simulink model "simli_wdc_wWT"  (R2023b)
settings: Solver=VariableStepAuto  StartTime=0.0  StopTime=10  RelTol=1e-3
undefined symbols (not defined in the file or in its folder): A_s_denom, A_s_num, c_f, C_hv_km, Cagg, Cbase1v, Cbase_hv, Cbase_mv, delta_vsc_0, G_dc_denom, G_dc_num, H_gen, H_vsm, i_d_vsc, i_q_vsc, Ibase_hv, Ibase_mv, k_d_vsm, k_p_p_vsm, k_p_q_vsm, k_vc, ki, ki_q, kp, L_comp, l_f, l_grid, L_hv_km, l_t_ehvhv, l_t_hvmv, l_t_mvlv, Lagg, Lbase_hv, Lbase_mv, length_export, M_gr_denom, M_gr_num, mppt_gain, omega_nom, omega_WTR_0, omega_WTR_n, P_meas, P_t, phase_shift_test_state, phase_shifts, pie_export, Q_meas, r_f, r_grid, R_hv_km, r_sys, r_t_ehvhv, r_t_hvmv, r_t_mvlv, Ragg, Rd, rocof_slope, Rocof_test_state, T_dc_denom, T_dc_num ... (+21)
libraries: slpidlib x9, spsFirstOrderFilterLib x1, simulink x1, spsSampleandHoldLib x1, spspowerguiLib x1
(part 1 of 3)
settings Model: Creator=Martin Pedersen  LastModifiedBy=Martin Pedersen

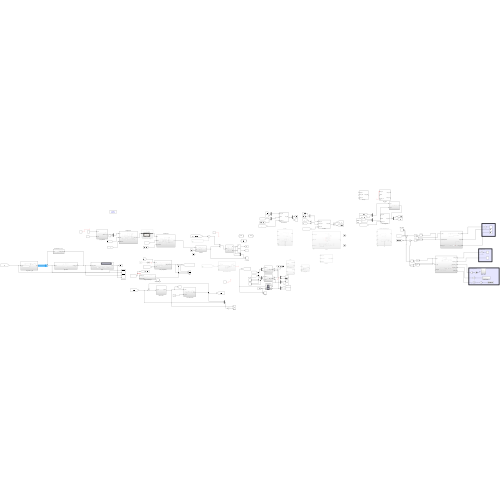
[thumbnail: Simulink's stored preview of the top-level diagram]
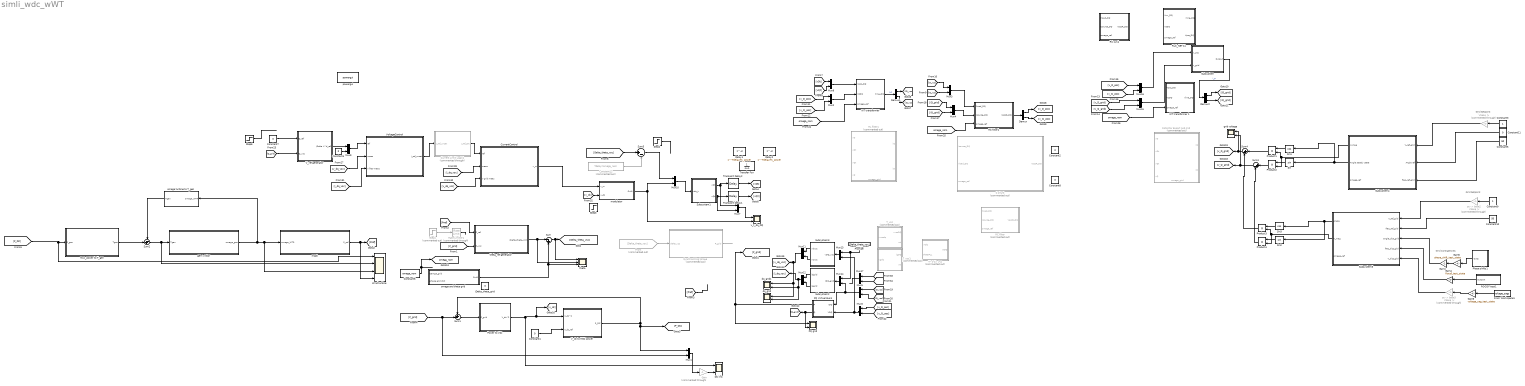
== system simli_wdc_wWT ==
  note: Grid Setpoint
  note: Grid Setpoint
  note: Grid Contigencies
  C shunt : Subsystem  Commented=on
  Collector Export and grid : Subsystem  Commented=on
      settings: PortSchema="{\"entries\":[{\"content\":{\"sides\":[{\"content\":{\"connectorIds\":[\"In1\",\"In2\",\"In3\",\"In4\"]},\"type\":\"ConnectorPlacement.EquallySpacedRectSide\",\"uuid\":\"57ad71d1-5664-4b35-a20c-d71f7e1cdc47\"},{\"content\":{\"connectorIds\":[\"Out1\",\"Out2\"],\"side\":\"RIGHT\"},\"type\":\"ConnectorPlacement.EquallySpacedRectSide\",\"uuid\":\"8101605d-eedb-4c26-847d-0cc0ce629d60\"},{\"content\":{\"side\":\"TOP\"},\"type\":\"ConnectorPlacement.EquallySpacedRectSide\",\"uuid\":\"2627b00b-24a5-469a-be2d-9c3c8a1d2080\"},{\"content\":{\"connectorIds\":[\"In5\"],\"side\":\"BOTTOM\"},\"type\":\"ConnectorPlacement.EquallySpacedRectSide\",\"uuid\":\"fe553db7-7727-4a02-b1e7-5aedfb7840ee\"}]},\"type\":\"ConnectorPlacement.EquallySpacedConnector\",\"uuid\":\"f40200c8-ad5b-428c-8a4e-7641595b86c4\"}],\"packageUris\":[\"http://schema.mathworks.com/mf0/Connector/R2020b\"],\"version\":\"1.0\"}"
  Constant{1..2,7..8,11} (5 alike) : Constant  Value=0
  Constant10 : Constant  Value=50
  Constant12 : Constant  Commented=on  Value=Tdelay*omega_nom
  Constant3 : Constant
  Constant4 : Constant  Value=0  SampleTime=Ts_power
  Constant5 : Constant  Value=50
  Constant6 : Constant  Value=omega_nom
  Constant9 : Constant
  Current Limit Logic1 : Subsystem  Commented=through
  CurrentControl : Subsystem
  DC link : Scope  NumInputPorts=2
  Delay1 : Delay  DelayLength=Tdelay/Ts_power
  Delay2 : Delay  DelayLength=Tdelay/Ts_power
  Demux : Demux  Outputs=2
  Demux1 : Demux  Outputs=2
  Demux2 : Demux  Outputs=2
  From : From  Commented=on  GotoTag=Delta_theta_vsc
  From Workspace1 : FromWorkspace  VariableName=voltage_sags
  Gain : Gain  Commented=through  Gain=-1
  Gain1 : Gain  Gain=-1
  Gain4 : Gain  Gain=Rocof_test_state
  Gain5 : Gain  Gain=phase_shift_test_state
  Gain6 : Gain  Gain=voltage_sag_test_state
  Mux{1..17} (17 alike) : Mux  Inputs=2
  PQ Virtual Bus1 : Subsystem
  PQ grid : Scope  NumInputPorts=2
  Phase shifts1 : Subsystem
  Power to Vdc : Subsystem
  Product{1..4} (4 alike) : Product
  RC filter : Subsystem  Commented=on  mask{Csource=c_f/omega_nom, Rd=0, VD0=1, VQ0=0}
      mask prompts: Csource "Net Capacitance"; Rd "Rdamp"
      mask help:
      | PI network, capacitance to enter is total.
      | Left and right current as input. Left and right voltage as output
      mask init:
      | inv_Csource=1/Csource;
      mask TypeOptions Csource: 8/Gain
      mask TypeOptions Rd: 1/Gain | 2/Gain
      mask TypeOptions VD0: VcpdR_int/InitialCondition
      mask TypeOptions VQ0: VcpqR_int/InitialCondition
  RC filter1 : Subsystem  mask{Csource=(c_f)/omega_nom, Rd=0, VD0=0, VQ0=0}
      mask prompts: Csource "Net Capacitance"; Rd "Rdamp"
      mask help:
      | PI network, capacitance to enter is total.
      | Left and right current as input. Left and right voltage as output
      mask init:
      | inv_Csource=1/Csource;
      mask TypeOptions Csource: 8/Gain
      mask TypeOptions Rd: 1/Gain | 2/Gain
      mask TypeOptions VD0: VcpdR_int/InitialCondition
      mask TypeOptions VQ0: VcpqR_int/InitialCondition
  RC sys1 : Subsystem  mask{Csource=(C_hv_km*length_export/Cbase_hv)/omega_nom, Rd=0.0001, VD0=0, VQ0=0}
      mask prompts: Csource "Net Capacitance"; Rd "Rdamp"
      mask help:
      | PI network, capacitance to enter is total.
      | Left and right current as input. Left and right voltage as output
      mask init:
      | inv_Csource=1/Csource;
      mask TypeOptions Csource: 8/Gain
      mask TypeOptions Rd: 1/Gain | 2/Gain
      mask TypeOptions VD0: VcpdR_int/InitialCondition
      mask TypeOptions VQ0: VcpqR_int/InitialCondition
  RL filter1 : Subsystem  Commented=on
      settings: PortSchema="{\"entries\":[{\"content\":{\"sides\":[{\"content\":{\"connectorIds\":[\"In1\",\"In2\",\"In3\",\"In4\"]},\"type\":\"ConnectorPlacement.EquallySpacedRectSide\",\"uuid\":\"57ad71d1-5664-4b35-a20c-d71f7e1cdc47\"},{\"content\":{\"connectorIds\":[\"Out1\",\"Out2\"],\"side\":\"RIGHT\"},\"type\":\"ConnectorPlacement.EquallySpacedRectSide\",\"uuid\":\"8101605d-eedb-4c26-847d-0cc0ce629d60\"},{\"content\":{\"side\":\"TOP\"},\"type\":\"ConnectorPlacement.EquallySpacedRectSide\",\"uuid\":\"2627b00b-24a5-469a-be2d-9c3c8a1d2080\"},{\"content\":{\"connectorIds\":[\"In5\"],\"side\":\"BOTTOM\"},\"type\":\"ConnectorPlacement.EquallySpacedRectSide\",\"uuid\":\"fe553db7-7727-4a02-b1e7-5aedfb7840ee\"}]},\"type\":\"ConnectorPlacement.EquallySpacedConnector\",\"uuid\":\"f40200c8-ad5b-428c-8a4e-7641595b86c4\"}],\"packageUris\":[\"http://schema.mathworks.com/mf0/Connector/R2020b\"],\"version\":\"1.0\"}"
  RLC_NET 11 : Subsystem  mask{Csource=(C_hv_km*length_export/pie_export/Cbase_hv)/omega_nom, Rsource=(R_hv_km*length_export/pie_export)/Zbase_hv, Lsource=(L_hv_km*length_export/pie_export/Lbase_hv)/omega_nom}
      mask prompts: Csource "line capacitance 1 side"; Rsource "Line resistance"; Lsource "line inductance"
      mask help:
      | RL with C terminations on right,
      | Left Voltage  and Right current input, Right voltage and left current output
      mask init:
      | inv_Csource=1/Csource;
      | inv_Lsource=1/Lsource;
      mask TypeOptions Csource: 8/Gain
      mask TypeOptions Rsource: 2/Gain | 3/Gain
      mask TypeOptions Lsource: 7/Gain
  ROCOF test1 : Subsystem
  Rate Limiter1 : RateLimiter  Commented=through  SampleTimeMode=inherited
  Sin : Trigonometry
  Sin1 : Trigonometry  Operator=cos
  Sin2 : Trigonometry
  Sin3 : Trigonometry  Operator=cos
  Step1 : Step  Commented=on  After=0.1  SampleTime=Ts_power
  Step2 : Step  Time=5  After=0  SampleTime=Ts_power
  Step3 : Step  Time=5  After=0  SampleTime=Ts_power
  Step6 : Step  After=0.1  SampleTime=Ts_power
  Subsystem : Subsystem
  Subsystem1 : Subsystem
  Subsystem2 : Subsystem
  Subsystem3 : Subsystem
  Subsystem4 : Subsystem
  Subsystem5 : Subsystem
  Sum : Sum  Inputs=|-+
  Sum1 : Sum  Inputs=+-|
  Sum2 : Sum  Inputs=-+|
  Sum3 : Sum  Inputs=|+-
  Sum4 : Sum  Inputs=|+-
  Sum5 : Sum  Inputs=|+-
  Synchronizing torque : Subsystem  Commented=on
  "T^{-1}_vsc" : Subsystem  Commented=on
  T_vsc : Subsystem  Commented=on  AncestorBlock=powerlib_meascontrol/Transformations/dq0 to Alpha-Beta-Zero/Subsystem1
  T_vsc1 : Subsystem  Commented=on  AncestorBlock=powerlib_meascontrol/Transformations/dq0 to Alpha-Beta-Zero/Subsystem1
  Transfer Fcn : TransferFcn  Denominator=[1 1]
  Transport Delay1 : TransportDelay  DelayTime=Tdelay/4  BufferSize=3560000  TransDelayFeedthrough=on
  Transport Delay2 : TransportDelay  DelayTime=Tdelay/4  BufferSize=3560000  TransDelayFeedthrough=on
  V_dc to MSC power : Subsystem
  V_ref generator : Subsystem
  VoltageControl : Subsystem
  "WT transformer " : Subsystem  mask{Rsource=r_f, Lsource=l_f/omega_nom}
      mask prompts: Rsource "Line resistance"; Lsource "line inductance"
      mask help:
      | RLV_NET is an 3 phase series RL with no virtual resistance termination,
      | 2 voltages as inputs and 1 current output
      mask init:
      | inv_Lsource=1/Lsource;
      mask TypeOptions Rsource: 2/Gain | 3/Gain
      mask TypeOptions Lsource: 7/Gain
  WT transformer 1 : Subsystem  mask{Rsource=r_sys, Lsource=x_sys/omega_nom}
      mask prompts: Rsource "Line resistance"; Lsource "line inductance"
      mask help:
      | RLV_NET is an 3 phase series RL with no virtual resistance termination,
      | 2 voltages as inputs and 1 current output
      mask init:
      | inv_Lsource=1/Lsource;
      mask TypeOptions Rsource: 2/Gain | 3/Gain
      mask TypeOptions Lsource: 7/Gain
  Wind turbine : Scope  NumInputPorts=4
  \Delta_theta_grid : Constant  Value=0
  dq_grid : Scope  NumInputPorts=2
  dq_grid1 : Scope  NumInputPorts=2
  gen->rotor : Subsystem
  grid voltage : Scope  NumInputPorts=2
  modulator : Subsystem
  mppt : Subsystem
  msc_power to T_gen : Subsystem
  omega and theta grid : Subsystem
  omega turbine to T_gen : Subsystem
  powergui : spspowerguiLib/powergui  Priority=1  SimulationMode=Discrete  SampleTime=Ts_power  frequency=60  Iterations=50  frequencyindice=60  Pbase=100e6  ErrMax=1e-4  UnitsV=kV  UnitsW=MW  buscounter=0  FunctionMessages=off  echomessages=off  EnableUseOfTLC=off  CurrentSourceSwitches=off  DisableSnubberDevices=off  DisableRonSwitches=off  DisableVfSwitches=off  DisplayEquations=off  AutomaticDiscreteSolvers=off  SolverType=Tustin/Backward Euler (TBE)  Interpol=off  ExternalGateDelay=off  methode=off  Ts=100  x0status=blocks  SPID=on  SwTol=0  HookPort=off  NonlinearTolerance=1e-4  nMaxIteration=100  ContinueOnMaxIteration=off  RestoreLinks=warning  ResistiveCurrentMeasurement=off  Frange=[0:2:500]  Ylog=off  Xlog=on  ShowGrid=off  save=off  variable=ZData  structure=0  ZoomFFT=off  StartTime=0.0  cycles=1  DisplayStyle=1  fundamental=60  FreqAxis=off  MaxFrequency=1000  frequencyindicesteady=1  RmsSteady=1  display=off
  "pu -> base" : Gain  Commented=through  Gain=Vbase_lv
  "pu -> base2" : Gain  Commented=through  Gain=Vbase_lv
  "pu -> base3" : Gain  Commented=through  Gain=Vbase_lv
  theta : Scope  NumInputPorts=3
  theta_ref generator : Subsystem
  v_t_dq_DQ : Scope  NumInputPorts=2
  tag scope: omega_nom=global
  wires:
  theta_ref generator/1(\Delta_theta_vsm) -> theta/2, Sum/1
  omega and theta grid/1(Out1) -> Sum/2, theta/3
  Sum/1 -> theta/1, [Delta_theta_vsc]
  V_ref generator/1(\Delta V^d_ref) -> Mux9/1
  From/1 -> Synchronizing torque/1(delta_vsc)
  [P_grid] -> theta_ref generator/2(P_vsc)
  [Pref] -> theta_ref generator/1(P_ref)
  [Pref] -> ?
  gen->rotor/1(omega_gen) -> omega turbine to T_gen/1(omega_WTR), Wind turbine/3, mppt/1(omega_WTR)
  Power to Vdc/1(V_dc^2) -> [v_dc], V_dc to MSC power/1(V_dc^2), DC link/1
  V_dc to MSC power/1(P_DC) -> Mux1/1, [P_DC], Sum1/1
  Sum1/1 -> Power to Vdc/1(P_grid)
  [P_grid] -> Mux1/2, Sum1/2
  Mux1/1 -> Gain/1
  Sum2/1 -> Wind turbine/2, gen->rotor/1(Tgen)
  msc_power to T_gen/1(Tgen) -> Sum2/2
  omega turbine to T_gen/1(Tgen) -> Sum2/1
  [P_DC] -> Wind turbine/1, msc_power to T_gen/1(P_gen)
  mppt/1(P_ref) -> Wind turbine/4, [Pref]
  Constant1/1 -> V_dc to MSC power/2(V_dc_ref)
  Step1/1 -> Rate Limiter1/1
  Gain/1 -> DC link/2
  Step2/1 -> ?
  Mux10/1 -> Subsystem1/1(vdq_t)
  [omega_nom] -> "WT transformer "/3(omega_ref)
  [vDt] -> Mux8/1
  [vQt] -> Mux8/2
  Demux1/1 -> [iD_vsc]
  Demux1/2 -> [iQ_vsc]
  [iQ_vsc] -> Mux3/2
  [iD_vsc] -> Mux3/1
  RC filter1/1(VpccR_DQ) -> Demux/1
  Demux/1 -> [v_D_poc]
  Demux/2 -> [v_Q_poc]
  [v_D_poc] -> Mux2/1
  [v_Q_poc] -> Mux2/2
  [v_Q_grid] -> Mux15/2
  [v_D_grid] -> Mux15/1
  Demux2/2 -> [iQ_grid]
  Demux2/1 -> [iD_grid]
  [v_Q_poc] -> Mux16/2
  [v_D_poc] -> Mux16/1
  [omega_nom] -> WT transformer 1/3(omega_ref)
  [iQ_grid] -> Mux4/2
  [iD_grid] -> Mux4/1
  [iQ_vsc] -> Mux5/2
  [iD_vsc] -> Mux5/1
  [v_Q_poc] -> Mux6/2
  [v_D_poc] -> Mux6/1
  PQ Virtual Bus1/2(Q) -> PQ grid/2, [Q_grid]
  [Q_grid] -> V_ref generator/2(Q_vsc)
  Step6/1 -> ?
  Mux7/1 -> v_t_dq_DQ/1
  [Delta_theta_vsc] -> Sum5/1
  Mux6/1 -> Mux13/2, PQ Virtual Bus1/2(VDQ)
  Mux4/1 -> RC filter1/2("Isource_DQ ")
  Mux3/1 -> RC filter1/1(Iload_DQ)
  [omega_nom] -> RC filter1/3(omega_ref)
  Constant6/1 -> [omega_nom]
  Synchronizing torque/1(P_grid) -> ?
  Rate Limiter1/1 -> ?
  VoltageControl/1(I_ref_unsat) -> Current Limit Logic1/1(I_ref_unsat)
  Current Limit Logic1/1(I_ref_sat) -> CurrentControl/1(ref)
  Constant4/1 -> Mux9/2
  Mux9/1 -> VoltageControl/1(ref)
  Mux5/1 -> Mux14/2, PQ Virtual Bus1/1(IDQ)
  Subsystem3/1(vdvsc) -> Mux11/1
  Subsystem3/2(vqvsc) -> Mux11/2
  Subsystem2/1(idgrid) -> Mux12/1
  Subsystem2/2(iqgrid) -> Mux12/2
  Mux12/1 -> dq_grid1/2, dq_grid/2, [i_dq_vsc]
  Mux11/1 -> dq_grid1/1, dq_grid/1, [v_dq_vsc]
  [v_dq_vsc] -> VoltageControl/2(meas)
  [i_dq_vsc] -> CurrentControl/2(meas)
  Mux14/1 -> Subsystem2/1(iDQ_grid)
  Mux13/1 -> Subsystem3/1(vDQ_vsc)
  [Delta_theta_vsc] -> Mux14/1, Mux13/1
  [v_dq_vsc] -> CurrentControl/3(V grid meas)
  [i_dq_vsc] -> VoltageControl/3(I filter meas)
  Constant7/1 -> V_ref generator/1(Q_ref)
  Mux2/1 -> "WT transformer "/2("VsDQ ")
  Mux8/1 -> "WT transformer "/1(Vpcc_DQ)
  "WT transformer "/1(Iline_DQ) -> Demux1/1  "i_o"
  Mux15/1 -> Subsystem/2(v_grid)
  Mux16/1 -> Subsystem/1(v_pcc)
  Subsystem/1(Output) -> Demux2/1  "i_o"
  [v_dc] -> modulator/2(v_dc)
  modulator/1(Out1) -> Mux10/2, v_t_dq_DQ/2
  Subsystem4/2(Angle steady state) -> Sin1/1, Sin/1
  "pu -> base"/1 -> Subsystem4/1(V_ref_grid)
  Sin1/1 -> Product1/1
  Sin2/1 -> Product4/1
  Subsystem4/1(V_mag) -> Product1/2, Product2/2
  Product3/1 -> Sum4/2
  From Workspace1/1 -> Gain6/1
  Gain4/1 -> Subsystem5/4(freq_dist_grid)
  Subsystem5/1(Angle) -> Sin2/1, Sin3/1
  Sum3/1 -> [v_Q_grid], grid voltage/2
  Gain1/1 -> Subsystem5/3(angle_dist_grid)
  Gain6/1 -> "pu -> base3"/1
  Constant9/1 -> "pu -> base2"/1
  "pu -> base2"/1 -> Subsystem5/1(V_ref_grid)
  ROCOF test1/1(Outport) -> Gain4/1
  Sin3/1 -> Product3/1
  Sin/1 -> Product2/1
  "pu -> base3"/1 -> Subsystem5/5(V_dist_grid)
  Subsystem5/2(V_mag) -> Product4/2, Product3/2
  Product2/1 -> Sum3/1
  Constant5/1 -> Subsystem4/3(freq_ref_grid)
  Constant10/1 -> Subsystem5/2(freq_ref_grid)
  Product1/1 -> Sum4/1
  Product4/1 -> Sum3/2
  Constant11/1 -> Subsystem4/2(Angle ref)
  Gain5/1 -> Gain1/1
  Phase shifts1/1(Out2) -> Gain5/1
  Sum4/1 -> grid voltage/1, [v_D_grid]
  Constant3/1 -> "pu -> base"/1
  Subsystem1/1(vDt) -> Transport Delay2/1, Mux7/1
  Subsystem1/2(vQt) -> Transport Delay1/1, Mux7/2
  Constant12/1 -> Sum5/2
  Sum5/1 -> Mux10/1
  CurrentControl/1(v_m) -> modulator/1(v_m)
  Transport Delay2/1 -> [vDt]
  Transport Delay1/1 -> [vQt]
  ? -> RLC_NET 11/1(Iinv_DQ)
  PQ Virtual Bus1/1(P) -> [P_grid], PQ grid/1
  Mux17/1 -> ?
  [iD_grid] -> Mux17/1
  [iQ_grid] -> Mux17/2

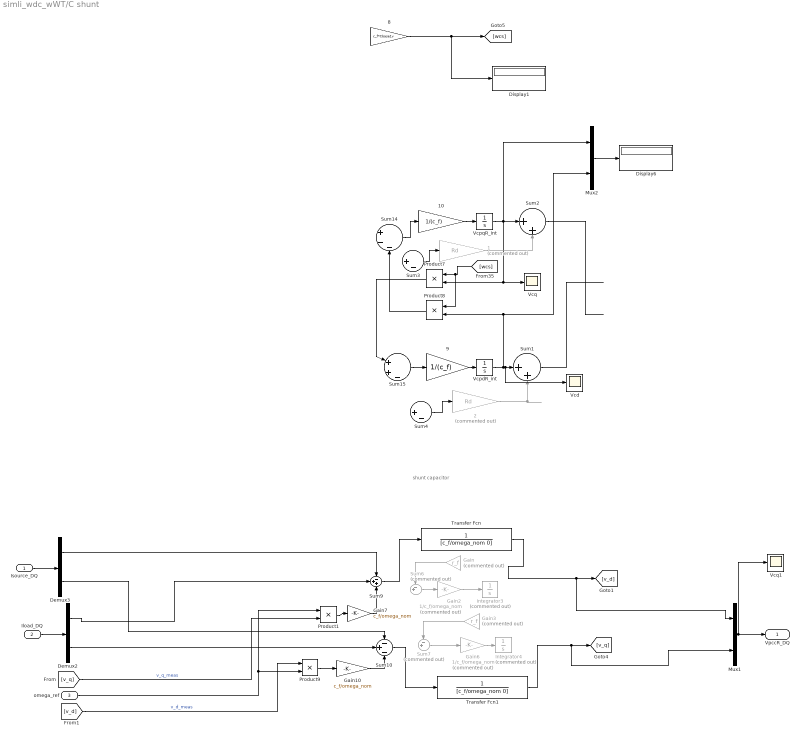
== system simli_wdc_wWT/C shunt ==
  note: shunt capacitor
  "Isource_DQ " : Inport
  Iload_DQ : Inport  Port=2
  omega_ref : Inport  Port=3
  1 : Gain  Commented=on  Gain=Rd
  10 : Gain  Gain=1/(c_f)
  2 : Gain  Commented=on  Gain=Rd
  8 : Gain  Gain=c_f*Cbase1v
  9 : Gain  Gain=1/(c_f)
  Demux2 : Demux  Outputs=2
  Demux3 : Demux  Outputs=2
  Display1 : Display
  Display6 : Display
  Gain : Gain  Commented=on  Gain=r_f
  Gain10 : Gain  Gain=c_f/omega_nom
  Gain2 : Gain  Commented=on  Gain=1/c_f/omega_nom
  Gain3 : Gain  Commented=on  Gain=r_f
  Gain6 : Gain  Commented=on  Gain=1/c_f/omega_nom
  Gain7 : Gain  Gain=c_f/omega_nom
  Integrator3 : Integrator  Commented=on
  Integrator4 : Integrator  Commented=on
  Mux1 : Mux  Inputs=2
  Mux2 : Mux  Inputs=2
  Product{1,7..9} (4 alike) : Product
  Sum1 : Sum  Inputs=|++
  Sum10 : Sum  Inputs=-+-
  Sum14 : Sum  Inputs=|+--
  Sum15 : Sum  Inputs=|++-
  Sum2 : Sum  Inputs=|++
  Sum3 : Sum  Inputs=|+-
  Sum4 : Sum  Inputs=|+-
  Sum6 : Sum  Commented=on  Inputs=-+|
  Sum7 : Sum  Commented=on  Inputs=-+|
  Sum9 : Sum  Inputs=-++
  Transfer Fcn : TransferFcn  Denominator=[c_f/omega_nom 0]
  Transfer Fcn1 : TransferFcn  Denominator=[c_f/omega_nom 0]
  Vcd : Scope
  VcpdR_int : Integrator  UpperSaturationLimit=50  LowerSaturationLimit=-1000
  VcpqR_int : Integrator  UpperSaturationLimit=50  LowerSaturationLimit=-1000
  Vcq : Scope
  Vcq1 : Scope
  VpccR_DQ : Outport  VectorParamsAs1DForOutWhenUnconnected=off
  wires:
  ? -> Sum15/2, Sum4/1
  VcpqR_int/1 -> Vcq/1, Product7/2, Sum2/1, Mux2/1
  1/1 -> Sum2/2
  2/1 -> Sum1/2
  Sum15/1 -> 9/1
  Product8/1 -> Sum14/3
  Sum14/1 -> 10/1
  8/1 -> Display1/1, [wcs]
  ? -> Sum15/3, Sum4/2
  Product7/1 -> Sum15/1
  ? -> 8/1
  ? -> Sum14/1, Sum3/1
  [wcs] -> Product8/1, Product7/1
  9/1 -> VcpdR_int/1
  ? -> Sum14/2, Sum3/2
  Sum3/1 -> 1/1
  10/1 -> VcpqR_int/1
  Mux2/1 -> Display6/1
  Sum4/1 -> 2/1
  Sum1/1 -> ?
  Sum2/1 -> ?
  VcpdR_int/1 -> Vcd/1, Sum1/1, Product8/2, Mux2/2
  Gain6/1 -> Integrator4/1
  omega_ref/1 -> Product9/2, Product1/1
  Demux3/1 -> Sum9/1
  Gain/1 -> Sum6/1
  Gain10/1 -> Sum10/3
  Sum7/1 -> Gain6/1
  Gain7/1 -> Sum9/3
  [v_d] -> Product9/1  "v_d_meas"
  Sum6/1 -> Gain2/1
  Product1/1 -> Gain7/1
  Demux2/2 -> Sum10/2
  Gain3/1 -> Sum7/1
  Transfer Fcn1/1 -> Mux1/2, [v_q]
  Demux3/2 -> Sum10/1
  [v_q] -> Product1/2  "v_q_meas"
  Transfer Fcn/1 -> Mux1/1, [v_d]
  Sum10/1 -> Transfer Fcn1/1
  Gain2/1 -> Integrator3/1
  Sum9/1 -> Transfer Fcn/1
  Demux2/1 -> Sum9/2
  Product9/1 -> Gain10/1
  Iload_DQ/1 -> Demux2/1
  "Isource_DQ "/1 -> Demux3/1
  Mux1/1 -> Vcq1/1, VpccR_DQ/1

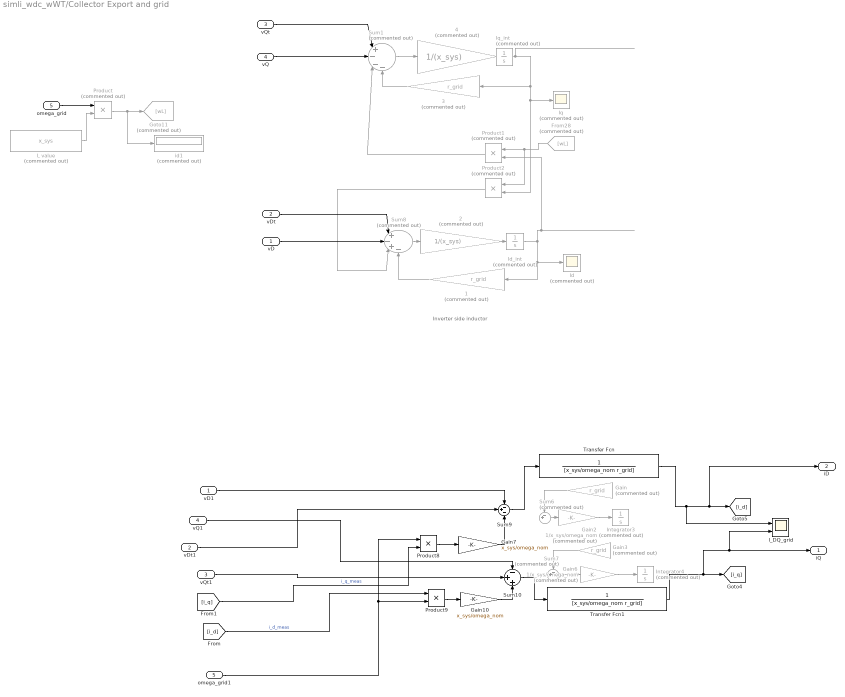
== system simli_wdc_wWT/Collector Export and grid ==
  note: Inverter side inductor
  vD : Inport
  vDt : Inport  Port=2
  vQt : Inport  Port=3
  vQ : Inport  Port=4
  omega_grid : Inport  Port=5
  1 : Gain  Commented=on  Gain=r_grid
  2 : Gain  Commented=on  Gain=1/(x_sys)
  3 : Gain  Commented=on  Gain=r_grid
  4 : Gain  Commented=on  Gain=1/(x_sys)
  From28 : From  Commented=on  GotoTag=wL
  Gain : Gain  Commented=on  Gain=r_grid
  Gain10 : Gain  Gain=x_sys/omega_nom
  Gain2 : Gain  Commented=on  Gain=1/x_sys/omega_nom
  Gain3 : Gain  Commented=on  Gain=r_grid
  Gain6 : Gain  Commented=on  Gain=1/x_sys/omega_nom
  Gain7 : Gain  Gain=x_sys/omega_nom
  Goto11 : Goto  Commented=on  GotoTag=wL
  I_DQ_grid : Scope  NumInputPorts=2
  Id : Scope  Commented=on
  Id_int : Integrator  Commented=on  UpperSaturationLimit=50  LowerSaturationLimit=-1000
  Integrator3 : Integrator  Commented=on
  Integrator4 : Integrator  Commented=on
  Iq : Scope  Commented=on
  Iq_int : Integrator  Commented=on  UpperSaturationLimit=50  LowerSaturationLimit=-1000
  L value : Constant  Commented=on  Value=x_sys  SampleTime=-1
  Product : Product  Commented=on
  Product1 : Product  Commented=on
  Product2 : Product  Commented=on
  Product8 : Product
  Product9 : Product
  Sum1 : Sum  Commented=on  Inputs=|+---
  Sum10 : Sum  Inputs=-++
  Sum6 : Sum  Commented=on  Inputs=-+|
  Sum7 : Sum  Commented=on  Inputs=-+|
  Sum8 : Sum  Commented=on  Inputs=|+-+-
  Sum9 : Sum  Inputs=-+-
  Transfer Fcn : TransferFcn  Denominator=[x_sys/omega_nom r_grid]
  Transfer Fcn1 : TransferFcn  Denominator=[x_sys/omega_nom r_grid]
  id1 : Display  Commented=on
  omega_grid1 : InportShadow  Port=5
  vD1 : InportShadow
  vDt1 : InportShadow  Port=2
  vQ1 : InportShadow  Port=4
  vQt1 : InportShadow  Port=3
  iQ : Outport
  iD : Outport  Port=2
  wires:
  From28/1 -> Product2/1, Product1/1
  Id_int/1 -> 1/1, Id/1, Product1/2
  1/1 -> Sum8/4
  Product1/1 -> Sum1/3
  3/1 -> Sum1/4
  Sum1/1 -> 4/1
  2/1 -> Id_int/1
  Sum8/1 -> 2/1
  4/1 -> Iq_int/1
  Iq_int/1 -> Product2/2, Iq/1, 3/1
  Product2/1 -> Sum8/3
  vDt/1 -> Sum8/1
  vD/1 -> Sum8/2
  vQt/1 -> Sum1/1
  vQ/1 -> Sum1/2
  L value/1 -> Product/2
  Product/1 -> id1/1, Goto11/1
  omega_grid/1 -> Product/1
  Gain6/1 -> Integrator4/1
  vD1/1 -> Sum9/1
  Gain/1 -> Sum6/1
  Gain10/1 -> Sum10/3
  Sum7/1 -> Gain6/1
  Gain7/1 -> Sum9/3
  [i_d] -> Product9/1  "i_d_meas"
  Sum6/1 -> Gain2/1
  Product8/1 -> Gain7/1
  vQt1/1 -> Sum10/2
  Gain3/1 -> Sum7/1
  Transfer Fcn1/1 -> I_DQ_grid/2, iQ/1, [i_q]
  vQ1/1 -> Sum10/1
  [i_q] -> Product8/2  "i_q_meas"
  Transfer Fcn/1 -> I_DQ_grid/1, iD/1, [i_d]
  Sum10/1 -> Transfer Fcn1/1
  Sum9/1 -> Transfer Fcn/1
  vDt1/1 -> Sum9/2
  omega_grid1/1 -> Product8/1, Product9/2
  Gain2/1 -> Integrator3/1
  Product9/1 -> Gain10/1

== system simli_wdc_wWT/Current Limit Logic1 ==
  note: Circular Current limiter
  I_ref_unsat : Inport
  Abs1 : Abs
  Constant3 : Constant
  Constant4 : Constant  Value=1.2
  Demux6 : Demux  Outputs=2
  Demux7 : Demux  Outputs=[vect vect]
  Display3 : Display
  Divide : Product  Inputs=*/
  Divide1 : Product  Inputs=*/
  First-Order Filter1 : spsFirstOrderFilterLib/First-Order Filter  FilterType=Lowpass  Tc=0.002  Ts=0  Initialize=on  Vac_Init=[0, 0, 50]  Vdc_Init=0  PlotResponse=off  FreqRange="[0,  200,  1]"
  GreaterThan1 : RelationalOperator  Operator=>  OutDataTypeStr=boolean  RndMeth=Simplest  InputSameDT=off
  I_d_error2 : Scope  Commented=on
  I_d_error3 : Scope
  I_d_error5 : Scope  Commented=on
  Kip12 : Gain
  Kip13 : Gain  Gain=1/1.2
  Mux6 : Mux  Inputs=[vect vect]
  Real-Imag to Complex1 : RealImagToComplex
  Switch1 : Switch  Threshold=1  SaturateOnIntegerOverflow=off  InputSameDT=off
  Unit Delay2 : UnitDelay  InitialCondition=1  SampleTime=Ts_power  HasFrameUpgradeWarning=on
  Vmd2 : Display
  I_ref_sat : Outport
  wires:
  Mux6/1 -> I_ref_sat/1
  Divide1/1 -> Mux6/2
  Demux6/2 -> Real-Imag to Complex1/2
  Abs1/1 -> Kip13/1, I_d_error2/1, GreaterThan1/1
  Unit Delay2/1 -> Divide1/2, Divide/2
  Real-Imag to Complex1/1 -> Abs1/1
  Demux7/2 -> Divide1/1
  GreaterThan1/1 -> Switch1/2
  Demux6/1 -> Real-Imag to Complex1/1
  I_ref_unsat/1 -> Demux7/1, I_d_error5/1, Vmd2/1, First-Order Filter1/1
  Demux7/1 -> Divide/1
  Constant3/1 -> Switch1/3
  Kip13/1 -> Switch1/1
  Constant4/1 -> GreaterThan1/2
  Switch1/1 -> Kip12/1, I_d_error3/1
  Divide/1 -> Mux6/1
  Kip12/1 -> Display3/1, Unit Delay2/1
  First-Order Filter1/1 -> Demux6/1

== system simli_wdc_wWT/CurrentControl ==
  ref : Inport
  meas : Inport  Port=2
  V grid meas : Inport  Port=3
  Constant : Constant
  Demux : Demux  Outputs=[vect vect]
  Demux1 : Demux  Outputs=[vect vect]
  Demux2 : Demux  Outputs=[vect vect]
  Divide1 : Product  Inputs=**
  Divide2 : Product  Inputs=**
  Gain4 : Gain  Gain=l_f
  Gain5 : Gain  Gain=l_f
  Mux : Mux  Inputs=[vect vect]
  Mux1 : Mux  Inputs=3
  Mux2 : Mux  Inputs=3
  PID Controller : slpidlib/PID Controller  Commented=on  Controller=PI  Form=Ideal  TimeDomain=Continuous-time  UseExternalTs=off  SampleTime=-1  IntegratorMethod=Forward Euler  FilterMethod=Forward Euler  ControllerParametersSource=internal  P=kp  I=ki  UseKiTs=off  D=0  N=100  UseFilter=on  TunerSelectOption=Transfer Function Based (PID Tuner App)  InitialConditionSource=internal  InitialConditionForIntegrator=0  InitialConditionForFilter=0  DifferentiatorICPrevScaledInput=0  ExternalReset=none  TrackingMode=off  Kt=1  LimitOutput=off  SatLimitsSource=internal  UpperSaturationLimit=inf  LowerSaturationLimit=-inf  LinearizeAsGain=on  AntiWindupMode=none  Kb=1  LimitIntegrator=off  UpperIntegratorSaturationLimit=inf  LowerIntegratorSaturationLimit=-inf  POutMin=[]  POutMax=[]  IOutMin=[]  IOutMax=[]  DOutMin=[]  DOutMax=[]  NOutMin=[]  NOutMax=[]  SumOutMin=[]  SumOutMax=[]  SaturationOutMin=[]  SaturationOutMax=[]  PParamMin=[]  PParamMax=[]  IParamMin=[]  IParamMax=[]  DParamMin=[]  DParamMax=[]  NParamMin=[]  NParamMax=[]  KbParamMin=[]  KbParamMax=[]  KtParamMin=[]  KtParamMax=[]  KbOutMin=[]  KbOutMax=[]  KtOutMin=[]  KtOutMax=[]  IntegratorOutMin=[]  IntegratorOutMax=[]  FilterOutMin=[]  FilterOutMax=[]  SumI1OutMin=[]  SumI1OutMax=[]  SumI2OutMin=[]  SumI2OutMax=[]  SumI3OutMin=[]  SumI3OutMax=[]  SumI4OutMin=[]  SumI4OutMax=[]  SumDOutMin=[]  SumDOutMax=[]  DifferentiatorOutMin=[]  DifferentiatorOutMax=[]  FilterDiffOutCoefMin=[]  FilterDiffOutCoefMax=[]  ReciprocalOutMin=[]  ReciprocalOutMax=[]  SumDenOutMin=[]  SumDenOutMax=[]  SumNumOutMin=[]  SumNumOutMax=[]  DivideOutMin=[]  DivideOutMax=[]  UdiffTsProdOutMin=[]  UdiffTsProdOutMax=[]  NTsProdOutMin=[]  NTsProdOutMax=[]  UintegralTsProdOutMin=[]  UintegralTsProdOutMax=[]  UngainTsProdOutMin=[]  UngainTsProdOutMax=[]  ClampingZeroOutDataTypeStr=Inherit: Inherit via back propagation  ClampingZeroOutMin=[]  ClampingZeroOutMax=[]  FilterDenConstantOutDataTypeStr=Inherit: Inherit via back propagation  FilterDenConstantOutMin=[]  FilterDenConstantOutMax=[]  PCopyOutDataTypeStr=Inherit: Inherit via back propagation  PCopyOutMin=[]  PCopyOutMax=[]  NCopyOutDataTypeStr=Inherit: Inherit via back propagation  NCopyOutMin=[]  NCopyOutMax=[]  IntegratorContinuousStateAttributes=''  IntegratorStateMustResolveToSignalObject=off  IntegratorRTWStateStorageClass=Auto  FilterContinuousStateAttributes=''  FilterStateMustResolveToSignalObject=off  FilterRTWStateStorageClass=Auto  ParallelPVariant=Passthrough  IdealPVariant=InternalParameters  IVariant=InternalParameters  DVariant=Disabled  IntegratorVariant=Continuous  SatVariant=Disabled  AWVariant=Passthrough  PCopyVariant=Disabled  TRVariant=Disabled  FdbkBlocksVariant=Forward  IdealPFdbkVariant=Disabled  SatFdbkVariant=Disabled  DerivativeFilterVariant=Disabled  NVariant=Disabled  NCopyVariant=Disabled_SignalSpec  FilterICVariant=Disabled  IntegratorICVariant=InternalICs  ExternalResetVariant=Disabled  TRSumVariant=Passthrough  SumFdbkVariant=Disabled  SumVariant=Sum_PI  TsampFilterVariant=InternalTs  TsampNgainVariant=Passthrough  TsampIntegralVariant=Disabled_SignalSpec  ExternalSaturationOutDataTypeStr=Inherit: Same as second input
  PID Controller1 : slpidlib/PID Controller  Commented=on  Controller=PI  Form=Ideal  TimeDomain=Continuous-time  UseExternalTs=off  SampleTime=-1  IntegratorMethod=Forward Euler  FilterMethod=Forward Euler  ControllerParametersSource=internal  P=kp  I=ki  UseKiTs=off  D=0  N=100  UseFilter=on  TunerSelectOption=Transfer Function Based (PID Tuner App)  InitialConditionSource=internal  InitialConditionForIntegrator=0  InitialConditionForFilter=0  DifferentiatorICPrevScaledInput=0  ExternalReset=none  TrackingMode=off  Kt=1  LimitOutput=off  SatLimitsSource=internal  UpperSaturationLimit=inf  LowerSaturationLimit=-inf  LinearizeAsGain=on  AntiWindupMode=none  Kb=1  LimitIntegrator=off  UpperIntegratorSaturationLimit=inf  LowerIntegratorSaturationLimit=-inf  POutMin=[]  POutMax=[]  IOutMin=[]  IOutMax=[]  DOutMin=[]  DOutMax=[]  NOutMin=[]  NOutMax=[]  SumOutMin=[]  SumOutMax=[]  SaturationOutMin=[]  SaturationOutMax=[]  PParamMin=[]  PParamMax=[]  IParamMin=[]  IParamMax=[]  DParamMin=[]  DParamMax=[]  NParamMin=[]  NParamMax=[]  KbParamMin=[]  KbParamMax=[]  KtParamMin=[]  KtParamMax=[]  KbOutMin=[]  KbOutMax=[]  KtOutMin=[]  KtOutMax=[]  IntegratorOutMin=[]  IntegratorOutMax=[]  FilterOutMin=[]  FilterOutMax=[]  SumI1OutMin=[]  SumI1OutMax=[]  SumI2OutMin=[]  SumI2OutMax=[]  SumI3OutMin=[]  SumI3OutMax=[]  SumI4OutMin=[]  SumI4OutMax=[]  SumDOutMin=[]  SumDOutMax=[]  DifferentiatorOutMin=[]  DifferentiatorOutMax=[]  FilterDiffOutCoefMin=[]  FilterDiffOutCoefMax=[]  ReciprocalOutMin=[]  ReciprocalOutMax=[]  SumDenOutMin=[]  SumDenOutMax=[]  SumNumOutMin=[]  SumNumOutMax=[]  DivideOutMin=[]  DivideOutMax=[]  UdiffTsProdOutMin=[]  UdiffTsProdOutMax=[]  NTsProdOutMin=[]  NTsProdOutMax=[]  UintegralTsProdOutMin=[]  UintegralTsProdOutMax=[]  UngainTsProdOutMin=[]  UngainTsProdOutMax=[]  ClampingZeroOutDataTypeStr=Inherit: Inherit via back propagation  ClampingZeroOutMin=[]  ClampingZeroOutMax=[]  FilterDenConstantOutDataTypeStr=Inherit: Inherit via back propagation  FilterDenConstantOutMin=[]  FilterDenConstantOutMax=[]  PCopyOutDataTypeStr=Inherit: Inherit via back propagation  PCopyOutMin=[]  PCopyOutMax=[]  NCopyOutDataTypeStr=Inherit: Inherit via back propagation  NCopyOutMin=[]  NCopyOutMax=[]  IntegratorContinuousStateAttributes=''  IntegratorStateMustResolveToSignalObject=off  IntegratorRTWStateStorageClass=Auto  FilterContinuousStateAttributes=''  FilterStateMustResolveToSignalObject=off  FilterRTWStateStorageClass=Auto  ParallelPVariant=Passthrough  IdealPVariant=InternalParameters  IVariant=InternalParameters  DVariant=Disabled  IntegratorVariant=Continuous  SatVariant=Disabled  AWVariant=Passthrough  PCopyVariant=Disabled  TRVariant=Disabled  FdbkBlocksVariant=Forward  IdealPFdbkVariant=Disabled  SatFdbkVariant=Disabled  DerivativeFilterVariant=Disabled  NVariant=Disabled  NCopyVariant=Disabled_SignalSpec  FilterICVariant=Disabled  IntegratorICVariant=InternalICs  ExternalResetVariant=Disabled  TRSumVariant=Passthrough  SumFdbkVariant=Disabled  SumVariant=Sum_PI  TsampFilterVariant=InternalTs  TsampNgainVariant=Passthrough  TsampIntegralVariant=Disabled_SignalSpec  ExternalSaturationOutDataTypeStr=Inherit: Same as second input
  PID Controller2 : slpidlib/PID Controller  Controller=PI  Form=Ideal  TimeDomain=Continuous-time  UseExternalTs=off  SampleTime=-1  IntegratorMethod=Forward Euler  FilterMethod=Forward Euler  ControllerParametersSource=internal  P=0.06  I=1/0.0013  UseKiTs=off  D=0  N=100  UseFilter=on  TunerSelectOption=Transfer Function Based (PID Tuner App)  InitialConditionSource=internal  InitialConditionForIntegrator=0  InitialConditionForFilter=0  DifferentiatorICPrevScaledInput=0  ExternalReset=none  TrackingMode=off  Kt=1  LimitOutput=off  SatLimitsSource=internal  UpperSaturationLimit=inf  LowerSaturationLimit=-inf  LinearizeAsGain=on  AntiWindupMode=none  Kb=1  LimitIntegrator=off  UpperIntegratorSaturationLimit=inf  LowerIntegratorSaturationLimit=-inf  POutMin=[]  POutMax=[]  IOutMin=[]  IOutMax=[]  DOutMin=[]  DOutMax=[]  NOutMin=[]  NOutMax=[]  SumOutMin=[]  SumOutMax=[]  SaturationOutMin=[]  SaturationOutMax=[]  PParamMin=[]  PParamMax=[]  IParamMin=[]  IParamMax=[]  DParamMin=[]  DParamMax=[]  NParamMin=[]  NParamMax=[]  KbParamMin=[]  KbParamMax=[]  KtParamMin=[]  KtParamMax=[]  KbOutMin=[]  KbOutMax=[]  KtOutMin=[]  KtOutMax=[]  IntegratorOutMin=[]  IntegratorOutMax=[]  FilterOutMin=[]  FilterOutMax=[]  SumI1OutMin=[]  SumI1OutMax=[]  SumI2OutMin=[]  SumI2OutMax=[]  SumI3OutMin=[]  SumI3OutMax=[]  SumI4OutMin=[]  SumI4OutMax=[]  SumDOutMin=[]  SumDOutMax=[]  DifferentiatorOutMin=[]  DifferentiatorOutMax=[]  FilterDiffOutCoefMin=[]  FilterDiffOutCoefMax=[]  ReciprocalOutMin=[]  ReciprocalOutMax=[]  SumDenOutMin=[]  SumDenOutMax=[]  SumNumOutMin=[]  SumNumOutMax=[]  DivideOutMin=[]  DivideOutMax=[]  UdiffTsProdOutMin=[]  UdiffTsProdOutMax=[]  NTsProdOutMin=[]  NTsProdOutMax=[]  UintegralTsProdOutMin=[]  UintegralTsProdOutMax=[]  UngainTsProdOutMin=[]  UngainTsProdOutMax=[]  ClampingZeroOutDataTypeStr=Inherit: Inherit via back propagation  ClampingZeroOutMin=[]  ClampingZeroOutMax=[]  FilterDenConstantOutDataTypeStr=Inherit: Inherit via back propagation  FilterDenConstantOutMin=[]  FilterDenConstantOutMax=[]  PCopyOutDataTypeStr=Inherit: Inherit via back propagation  PCopyOutMin=[]  PCopyOutMax=[]  NCopyOutDataTypeStr=Inherit: Inherit via back propagation  NCopyOutMin=[]  NCopyOutMax=[]  IntegratorContinuousStateAttributes='cc_q'  IntegratorStateMustResolveToSignalObject=off  IntegratorRTWStateStorageClass=Auto  FilterContinuousStateAttributes=''  FilterStateMustResolveToSignalObject=off  FilterRTWStateStorageClass=Auto  ParallelPVariant=Passthrough  IdealPVariant=InternalParameters  IVariant=InternalParameters  DVariant=Disabled  IntegratorVariant=Continuous  SatVariant=Disabled  AWVariant=Passthrough  PCopyVariant=Disabled  TRVariant=Disabled  FdbkBlocksVariant=Forward  IdealPFdbkVariant=Disabled  SatFdbkVariant=Disabled  DerivativeFilterVariant=Disabled  NVariant=Disabled  NCopyVariant=Disabled_SignalSpec  FilterICVariant=Disabled  IntegratorICVariant=InternalICs  ExternalResetVariant=Disabled  TRSumVariant=Passthrough  SumFdbkVariant=Disabled  SumVariant=Sum_PI  TsampFilterVariant=InternalTs  TsampNgainVariant=Passthrough  TsampIntegralVariant=Disabled_SignalSpec  ExternalSaturationOutDataTypeStr=Inherit: Same as second input
  PID Controller3 : slpidlib/PID Controller  Controller=PI  Form=Ideal  TimeDomain=Continuous-time  UseExternalTs=off  SampleTime=-1  IntegratorMethod=Forward Euler  FilterMethod=Forward Euler  ControllerParametersSource=internal  P=0.06  I=1/0.0013  UseKiTs=off  D=0  N=100  UseFilter=on  TunerSelectOption=Transfer Function Based (PID Tuner App)  InitialConditionSource=internal  InitialConditionForIntegrator=0  InitialConditionForFilter=0  DifferentiatorICPrevScaledInput=0  ExternalReset=none  TrackingMode=off  Kt=1  LimitOutput=off  SatLimitsSource=internal  UpperSaturationLimit=inf  LowerSaturationLimit=-inf  LinearizeAsGain=on  AntiWindupMode=none  Kb=1  LimitIntegrator=off  UpperIntegratorSaturationLimit=inf  LowerIntegratorSaturationLimit=-inf  POutMin=[]  POutMax=[]  IOutMin=[]  IOutMax=[]  DOutMin=[]  DOutMax=[]  NOutMin=[]  NOutMax=[]  SumOutMin=[]  SumOutMax=[]  SaturationOutMin=[]  SaturationOutMax=[]  PParamMin=[]  PParamMax=[]  IParamMin=[]  IParamMax=[]  DParamMin=[]  DParamMax=[]  NParamMin=[]  NParamMax=[]  KbParamMin=[]  KbParamMax=[]  KtParamMin=[]  KtParamMax=[]  KbOutMin=[]  KbOutMax=[]  KtOutMin=[]  KtOutMax=[]  IntegratorOutMin=[]  IntegratorOutMax=[]  FilterOutMin=[]  FilterOutMax=[]  SumI1OutMin=[]  SumI1OutMax=[]  SumI2OutMin=[]  SumI2OutMax=[]  SumI3OutMin=[]  SumI3OutMax=[]  SumI4OutMin=[]  SumI4OutMax=[]  SumDOutMin=[]  SumDOutMax=[]  DifferentiatorOutMin=[]  DifferentiatorOutMax=[]  FilterDiffOutCoefMin=[]  FilterDiffOutCoefMax=[]  ReciprocalOutMin=[]  ReciprocalOutMax=[]  SumDenOutMin=[]  SumDenOutMax=[]  SumNumOutMin=[]  SumNumOutMax=[]  DivideOutMin=[]  DivideOutMax=[]  UdiffTsProdOutMin=[]  UdiffTsProdOutMax=[]  NTsProdOutMin=[]  NTsProdOutMax=[]  UintegralTsProdOutMin=[]  UintegralTsProdOutMax=[]  UngainTsProdOutMin=[]  UngainTsProdOutMax=[]  ClampingZeroOutDataTypeStr=Inherit: Inherit via back propagation  ClampingZeroOutMin=[]  ClampingZeroOutMax=[]  FilterDenConstantOutDataTypeStr=Inherit: Inherit via back propagation  FilterDenConstantOutMin=[]  FilterDenConstantOutMax=[]  PCopyOutDataTypeStr=Inherit: Inherit via back propagation  PCopyOutMin=[]  PCopyOutMax=[]  NCopyOutDataTypeStr=Inherit: Inherit via back propagation  NCopyOutMin=[]  NCopyOutMax=[]  IntegratorContinuousStateAttributes='cc_d'  IntegratorStateMustResolveToSignalObject=off  IntegratorRTWStateStorageClass=Auto  FilterContinuousStateAttributes=''  FilterStateMustResolveToSignalObject=off  FilterRTWStateStorageClass=Auto  ParallelPVariant=Passthrough  IdealPVariant=InternalParameters  IVariant=InternalParameters  DVariant=Disabled  IntegratorVariant=Continuous  SatVariant=Disabled  AWVariant=Passthrough  PCopyVariant=Disabled  TRVariant=Disabled  FdbkBlocksVariant=Forward  IdealPFdbkVariant=Disabled  SatFdbkVariant=Disabled  DerivativeFilterVariant=Disabled  NVariant=Disabled  NCopyVariant=Disabled_SignalSpec  FilterICVariant=Disabled  IntegratorICVariant=InternalICs  ExternalResetVariant=Disabled  TRSumVariant=Passthrough  SumFdbkVariant=Disabled  SumVariant=Sum_PI  TsampFilterVariant=InternalTs  TsampNgainVariant=Passthrough  TsampIntegralVariant=Disabled_SignalSpec  ExternalSaturationOutDataTypeStr=Inherit: Same as second input
  Step1 : Step  Before=1  SampleTime=0
  Step2 : Step  Before=1  SampleTime=0
  Sum1 : Sum  Inputs=|+-
  Sum2 : Sum  Inputs=+-|
  Sum4 : Sum  Inputs=++-
  Sum5 : Sum  Inputs=+++
  Transfer Fcn2 : TransferFcn  Commented=on  Denominator=[0.005 1]
  Transfer Fcn3 : TransferFcn  Commented=on  Denominator=[0.005 1]
  d-axis-control : Scope  NumInputPorts=3
  q-axis control : Scope  NumInputPorts=3
  v_m : Outport
  wires:
  Step2/1 -> Divide1/2
  Sum2/1 -> q-axis control/1, Divide1/1  "i_ref-i_meas"
  Mux2/1 -> q-axis control/2  "compensation"
  PID Controller3/1 -> Sum4/2, Mux1/2
  Step1/1 -> Divide2/2
  Divide2/1 -> PID Controller3/1
  Divide1/1 -> PID Controller2/1
  Transfer Fcn3/1 -> Mux2/1, Sum5/3
  ref/1 -> Demux/1
  Gain4/1 -> Mux2/3, Sum5/1
  Transfer Fcn2/1 -> Mux1/1, Sum4/1
  Gain5/1 -> Mux1/3, Sum4/3
  V grid meas/1 -> Demux2/1
  Mux1/1 -> d-axis-control/2
  Sum4/1 -> d-axis-control/3, Mux/1
  Demux2/2 -> Transfer Fcn3/1
  Sum5/1 -> q-axis control/3, Mux/2  "output"
  PID Controller2/1 -> Mux2/2, Sum5/2
  meas/1 -> Demux1/1
  Demux/1 -> Sum1/1
  Mux/1 -> v_m/1
  Demux/2 -> Sum2/1
  Demux1/1 -> Gain4/1, Sum1/2
  Demux1/2 -> Gain5/1, Sum2/2
  Sum1/1 -> Divide2/1, d-axis-control/1
  Demux2/1 -> Transfer Fcn2/1

== system simli_wdc_wWT/PQ Virtual Bus1 ==
  note: Linearized at op
  note: PQ Virtual bus
  IDQ : Inport
  VDQ : Inport  Port=2
  Constant : Constant  Value=P_meas
  Constant1 : Constant  Value=Q_meas
  Demux5 : Demux  Outputs=[vect vect]
  Demux6 : Demux  Outputs=[vect vect]
  Dot Product : DotProduct  OutDataTypeStr=Inherit: Inherit via internal rule
  Dot Product1 : DotProduct  OutDataTypeStr=Inherit: Inherit via internal rule
  Mux : Mux  Inputs=2
  Product{1,3..5} (4 alike) : Product  InputSameDT=on  SaturateOnIntegerOverflow=on  OutDataTypeStr=Inherit: Same as first input
  Sum : Sum  InputSameDT=on  SaturateOnIntegerOverflow=on  OutDataTypeStr=Inherit: Same as first input
  Sum1 : Sum  Inputs=+-  InputSameDT=on  SaturateOnIntegerOverflow=on  OutDataTypeStr=Inherit: Same as first input
  P : Outport
  Q : Outport  Port=2
  wires:
  Sum/1 -> ?
  VDQ/1 -> Mux/2, Demux6/1
  IDQ/1 -> Mux/1, Demux5/1
  Sum1/1 -> ?
  Product5/1 -> Sum1/2
  Product1/1 -> Sum1/1
  Demux6/2 -> Product4/1, Product1/1
  Demux5/1 -> Product1/2, Product3/1
  Demux6/1 -> Product3/2, Product5/1
  Product4/1 -> Sum/2
  Demux5/2 -> Product5/2, Product4/2
  Product3/1 -> Sum/1
  Constant/1 -> Dot Product/1
  Mux/1 -> Dot Product1/2, Dot Product/2
  Constant1/1 -> Dot Product1/1
  Dot Product1/1 -> Q/1
  Dot Product/1 -> P/1

== system simli_wdc_wWT/Phase shifts1 ==
  From Workspace : FromWorkspace  Commented=on  VariableName=phase_shifts  OutputAfterFinalValue=Setting to zero
  Gain : Gain  Gain=-1
  Step : Step  Time=phase_shifts(1,1)-40  After=phase_shifts(1,2)  SampleTime=0
  Step1 : Step  Time=phase_shifts(2,1)  After=phase_shifts(2,2)  SampleTime=0
  Step2 : Step  Time=phase_shifts(3,1)  After=phase_shifts(3,2)  SampleTime=0
  Sum1 : Sum  Inputs=++++
  theta_dist : Constant  Value=0
  Out2 : Outport
  wires:
  Sum1/1 -> Out2/1
  Step/1 -> Sum1/1
  Step2/1 -> Sum1/3
  From Workspace/1 -> ?
  Step1/1 -> Sum1/2
  theta_dist/1 -> Gain/1
  Gain/1 -> Sum1/4

== system simli_wdc_wWT/Power to Vdc ==
  P_grid : Inport
  DC_dynamics : TransferFcn  Numerator=-1*T_dc_num{1}  Denominator=T_dc_denom{1}  ContinuousStateAttributes='Delta_Vdc2'
  msc current control : TransferFcn  Commented=through  Denominator=[0.01 1]
  V_dc^2 : Outport
  wires:
  P_grid/1 -> msc current control/1
  DC_dynamics/1 -> V_dc^2/1
  msc current control/1 -> DC_dynamics/1

== system simli_wdc_wWT/RC filter ==
  note: shunt capacitor
  note: Left shunt capacitor
  Iload_DQ : Inport
  "Isource_DQ " : Inport  Port=2
  omega_ref : Inport  Port=3
  1 : Gain  Commented=on  Gain=Rd
  10 : Gain  Gain=inv_Csource
  2 : Gain  Commented=on  Gain=Rd
  8 : Gain  Gain=Csource
  9 : Gain  Gain=inv_Csource
  Demux2 : Demux  Outputs=2
  Demux3 : Demux  Outputs=2
  Display1 : Display
  Display6 : Display
  Mux1 : Mux  Inputs=2
  Mux2 : Mux  Inputs=2
  Product7 : Product
  Product8 : Product
  Sum1 : Sum  Inputs=|++
  Sum14 : Sum  Inputs=|+--
  Sum15 : Sum  Inputs=|++-
  Sum2 : Sum  Inputs=|++
  Sum3 : Sum  Inputs=|+-
  Sum4 : Sum  Inputs=|+-
  Vcd : Scope
  VcpdR_int : Integrator  InitialCondition=VD0  UpperSaturationLimit=50  LowerSaturationLimit=-1000
  VcpqR_int : Integrator  InitialCondition=VQ0  UpperSaturationLimit=50  LowerSaturationLimit=-1000
  Vcq : Scope
  VpccR_DQ : Outport  VectorParamsAs1DForOutWhenUnconnected=off
  wires:
  Sum4/1 -> 2/1
  Sum3/1 -> 1/1
  Mux2/1 -> Display6/1
  2/1 -> Vcd/1, Sum1/2
  1/1 -> Sum2/2
  Sum2/1 -> Mux1/2
  Sum1/1 -> Mux1/1
  VcpdR_int/1 -> Sum1/1, Product8/2, Mux2/2
  Demux3/1 -> Sum15/3, Sum4/2
  Demux3/2 -> Sum14/2, Sum3/2
  "Isource_DQ "/1 -> Demux3/1
  Iload_DQ/1 -> Demux2/1
  Demux2/2 -> Sum14/1, Sum3/1
  Demux2/1 -> Sum15/2, Sum4/1
  9/1 -> VcpdR_int/1
  Sum14/1 -> 10/1
  [wcs] -> Product8/1, Product7/1
  VcpqR_int/1 -> Vcq/1, Product7/2, Sum2/1, Mux2/1
  Product7/1 -> Sum15/1
  10/1 -> VcpqR_int/1
  Sum15/1 -> 9/1
  Product8/1 -> Sum14/3
  Mux1/1 -> VpccR_DQ/1
  8/1 -> Display1/1, [wcs]
  omega_ref/1 -> 8/1

== system simli_wdc_wWT/RC filter1 ==
  note: shunt capacitor
  note: Left shunt capacitor
  Iload_DQ : Inport
  "Isource_DQ " : Inport  Port=2
  omega_ref : Inport  Port=3
  1 : Gain  Gain=Rd
  10 : Gain  Gain=inv_Csource
  2 : Gain  Gain=Rd
  8 : Gain  Gain=Csource
  9 : Gain  Gain=inv_Csource
  Demux2 : Demux  Outputs=2
  Demux3 : Demux  Outputs=2
  Display1 : Display
  Display6 : Display
  Mux1 : Mux  Inputs=2
  Mux2 : Mux  Inputs=2
  Product7 : Product
  Product8 : Product
  Sum1 : Sum  Inputs=|++
  Sum14 : Sum  Inputs=|+--
  Sum15 : Sum  Inputs=|++-
  Sum2 : Sum  Inputs=|++
  Sum3 : Sum  Inputs=|+-
  Sum4 : Sum  Inputs=|+-
  Vcd : Scope
  VcpdR_int : Integrator  InitialCondition=VD0  UpperSaturationLimit=50  LowerSaturationLimit=-1000  ContinuousStateAttributes='Delta_v_vsc_D'
  VcpqR_int : Integrator  InitialCondition=VQ0  UpperSaturationLimit=50  LowerSaturationLimit=-1000  ContinuousStateAttributes='Delta_v_vsc_Q'
  Vcq : Scope
  VpccR_DQ : Outport  VectorParamsAs1DForOutWhenUnconnected=off
  wires:
  Sum4/1 -> 2/1
  Sum3/1 -> 1/1
  Mux2/1 -> Display6/1
  2/1 -> Vcd/1, Sum1/2
  1/1 -> Sum2/2
  Sum2/1 -> Mux1/2
  Sum1/1 -> Mux1/1
  VcpdR_int/1 -> Sum1/1, Product8/2, Mux2/2
  Demux3/1 -> Sum15/3, Sum4/2
  Demux3/2 -> Sum14/2, Sum3/2
  "Isource_DQ "/1 -> Demux3/1
  Iload_DQ/1 -> Demux2/1
  Demux2/2 -> Sum14/1, Sum3/1
  Demux2/1 -> Sum15/2, Sum4/1
  9/1 -> VcpdR_int/1
  Sum14/1 -> 10/1
  [wcs] -> Product8/1, Product7/1
  VcpqR_int/1 -> Vcq/1, Product7/2, Sum2/1, Mux2/1
  Product7/1 -> Sum15/1
  10/1 -> VcpqR_int/1
  Sum15/1 -> 9/1
  Product8/1 -> Sum14/3
  Mux1/1 -> VpccR_DQ/1
  8/1 -> Display1/1, [wcs]
  omega_ref/1 -> 8/1

== system simli_wdc_wWT/RC sys1 ==
  note: Left shunt capacitor
  note: shunt capacitor
  Iload_DQ : Inport
  "Isource_DQ " : Inport  Port=2
  omega_ref : Inport  Port=3
  1 : Gain  Gain=Rd
  10 : Gain  Gain=inv_Csource
  2 : Gain  Gain=Rd
  8 : Gain  Gain=Csource
  9 : Gain  Gain=inv_Csource
  Demux2 : Demux  Outputs=2
  Demux3 : Demux  Outputs=2
  Display1 : Display
  Display6 : Display
  Mux1 : Mux  Inputs=2
  Mux2 : Mux  Inputs=2
  Product7 : Product
  Product8 : Product
  Sum1 : Sum  Inputs=|++
  Sum14 : Sum  Inputs=|+--
  Sum15 : Sum  Inputs=|++-
  Sum2 : Sum  Inputs=|++
  Sum3 : Sum  Inputs=|+-
  Sum4 : Sum  Inputs=|+-
  Vcd : Scope
  VcpdR_int : Integrator  InitialCondition=VD0  UpperSaturationLimit=50  LowerSaturationLimit=-1000
  VcpqR_int : Integrator  InitialCondition=VQ0  UpperSaturationLimit=50  LowerSaturationLimit=-1000
  Vcq : Scope
  VpccR_DQ : Outport  VectorParamsAs1DForOutWhenUnconnected=off
  wires:
  8/1 -> [wcs], Display1/1
  Mux1/1 -> VpccR_DQ/1
  Product8/1 -> Sum14/3
  Sum15/1 -> 9/1
  10/1 -> VcpqR_int/1
  Product7/1 -> Sum15/1
  VcpqR_int/1 -> Mux2/1, Sum2/1, Product7/2, Vcq/1
  [wcs] -> Product7/1, Product8/1
  Sum14/1 -> 10/1
  9/1 -> VcpdR_int/1
  omega_ref/1 -> 8/1
  Demux2/1 -> Sum4/1, Sum15/2
  Demux2/2 -> Sum3/1, Sum14/1
  Iload_DQ/1 -> Demux2/1
  "Isource_DQ "/1 -> Demux3/1
  Demux3/2 -> Sum3/2, Sum14/2
  Demux3/1 -> Sum4/2, Sum15/3
  VcpdR_int/1 -> Mux2/2, Product8/2, Sum1/1
  Sum1/1 -> Mux1/1
  Sum2/1 -> Mux1/2
  1/1 -> Sum2/2
  2/1 -> Sum1/2
  Mux2/1 -> Display6/1
  Sum3/1 -> 1/1
  Sum4/1 -> 2/1

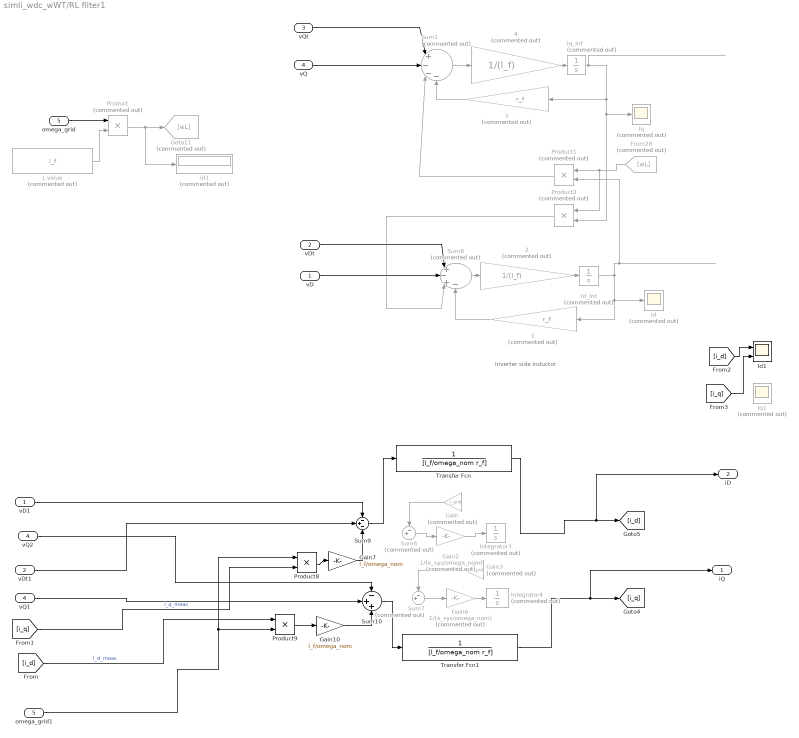
== system simli_wdc_wWT/RL filter1 ==
  note: Inverter side inductor
  vD : Inport
  vDt : Inport  Port=2
  vQt : Inport  Port=3
  vQ : Inport  Port=4
  omega_grid : Inport  Port=5
  1 : Gain  Commented=on  Gain=r_f
  2 : Gain  Commented=on  Gain=1/(l_f)
  3 : Gain  Commented=on  Gain=r_f
  4 : Gain  Commented=on  Gain=1/(l_f)
  From28 : From  Commented=on  GotoTag=wL
  Gain : Gain  Commented=on  Gain=r_grid
  Gain10 : Gain  Gain=l_f/omega_nom
  Gain2 : Gain  Commented=on  Gain=1/(x_sys/omega_nom)
  Gain3 : Gain  Commented=on  Gain=r_grid
  Gain6 : Gain  Commented=on  Gain=1/(x_sys/omega_nom)
  Gain7 : Gain  Gain=l_f/omega_nom
  Goto11 : Goto  Commented=on  GotoTag=wL
  Id : Scope  Commented=on
  Id1 : Scope  NumInputPorts=2
  Id_int : Integrator  Commented=on  UpperSaturationLimit=50  LowerSaturationLimit=-1000
  Integrator3 : Integrator  Commented=on
  Integrator4 : Integrator  Commented=on
  Iq : Scope  Commented=on
  Iq1 : Scope  Commented=on
  Iq_int : Integrator  Commented=on  UpperSaturationLimit=50  LowerSaturationLimit=-1000
  L value : Constant  Commented=on  Value=l_f  SampleTime=-1
  Product : Product  Commented=on
  Product1 : Product  Commented=on
  Product2 : Product  Commented=on
  Product8 : Product
  Product9 : Product
  Sum1 : Sum  Commented=on  Inputs=|+---
  Sum10 : Sum  Inputs=-++
  Sum6 : Sum  Commented=on  Inputs=-+|
  Sum7 : Sum  Commented=on  Inputs=-+|
  Sum8 : Sum  Commented=on  Inputs=|+-+-
  Sum9 : Sum  Inputs=-+-
  Transfer Fcn : TransferFcn  Denominator=[l_f/omega_nom r_f]
  Transfer Fcn1 : TransferFcn  Denominator=[l_f/omega_nom r_f]
  id1 : Display  Commented=on
  omega_grid1 : InportShadow  Port=5
  vD1 : InportShadow
  vDt1 : InportShadow  Port=2
  vQ1 : InportShadow  Port=4
  vQ2 : InportShadow  Port=4
  iQ : Outport
  iD : Outport  Port=2
  wires:
  omega_grid/1 -> Product/1
  Product/1 -> Goto11/1, id1/1
  L value/1 -> Product/2
  vQ/1 -> Sum1/2
  vQt/1 -> Sum1/1
  vD/1 -> Sum8/2
  vDt/1 -> Sum8/1
  Product2/1 -> Sum8/3
  Iq_int/1 -> 3/1, Iq/1, Product2/2
  4/1 -> Iq_int/1
  Sum8/1 -> 2/1
  2/1 -> Id_int/1
  Sum1/1 -> 4/1
  3/1 -> Sum1/4
  Product1/1 -> Sum1/3
  1/1 -> Sum8/4
  Id_int/1 -> Product1/2, Id/1, 1/1
  From28/1 -> Product1/1, Product2/1
  Sum6/1 -> Gain2/1
  Sum10/1 -> Transfer Fcn1/1
  Gain3/1 -> Sum7/1
  Sum7/1 -> Gain6/1
  vDt1/1 -> Sum9/2
  Product8/1 -> Gain7/1
  Transfer Fcn1/1 -> iQ/1, [i_q]
  Gain6/1 -> Integrator4/1
  Gain/1 -> Sum6/1
  Sum9/1 -> Transfer Fcn/1
  omega_grid1/1 -> Product8/1, Product9/2
  vQ1/1 -> Sum10/2
  Gain7/1 -> Sum9/3
  Product9/1 -> Gain10/1
  Gain10/1 -> Sum10/3
  [i_q] -> Product8/2  "i_q_meas"
  Transfer Fcn/1 -> iD/1, [i_d]
  [i_d] -> Product9/1  "i_d_meas"
  Gain2/1 -> Integrator3/1
  vD1/1 -> Sum9/1
  vQ2/1 -> Sum10/1
  [i_q] -> Id1/2
  [i_d] -> Id1/1

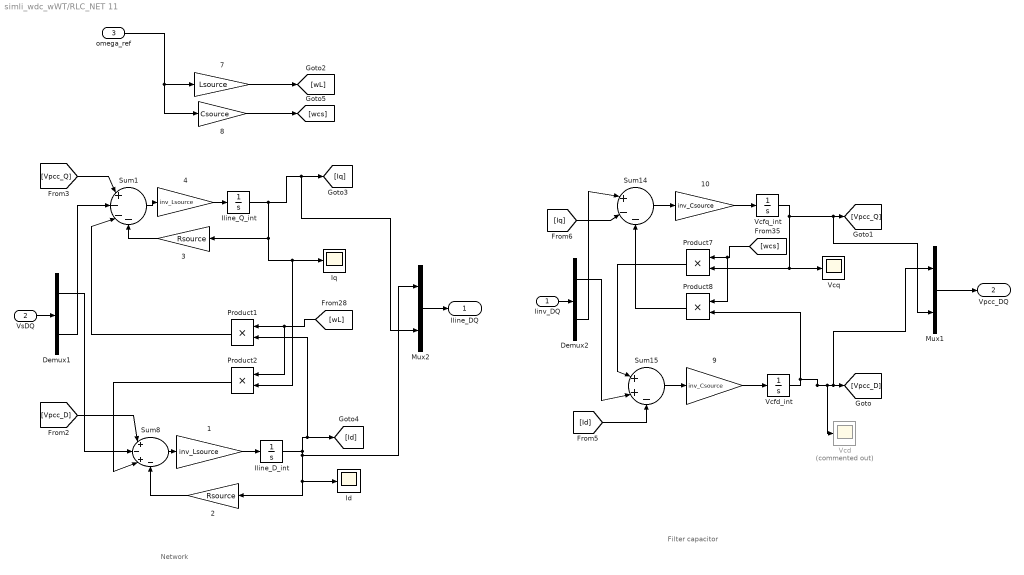
== system simli_wdc_wWT/RLC_NET 11 ==
  note: Network
  note: Filter capacitor
  Iinv_DQ : Inport
  "VsDQ " : Inport  Port=2
  omega_ref : Inport  Port=3
  1 : Gain  Gain=inv_Lsource
  10 : Gain  Gain=inv_Csource
  2 : Gain  Gain=Rsource
  3 : Gain  Gain=Rsource
  4 : Gain  Gain=inv_Lsource
  7 : Gain  Gain=Lsource
  8 : Gain  Gain=Csource
  9 : Gain  Gain=inv_Csource
  Demux1 : Demux  Outputs=2
  Demux2 : Demux  Outputs=2
  Id : Scope
  Iline_D_int : Integrator  UpperSaturationLimit=50  LowerSaturationLimit=-1000
  Iline_Q_int : Integrator  UpperSaturationLimit=50  LowerSaturationLimit=-1000
  Iq : Scope
  Mux1 : Mux  Inputs=2
  Mux2 : Mux  Inputs=2
  Product{1..2,7..8} (4 alike) : Product
  Sum1 : Sum  Inputs=|+---
  Sum14 : Sum  Inputs=|+--
  Sum15 : Sum  Inputs=|++-
  Sum8 : Sum  Inputs=|+-+-
  Vcd : Scope  Commented=on
  Vcfd_int : Integrator  UpperSaturationLimit=50  LowerSaturationLimit=-1000
  Vcfq_int : Integrator  UpperSaturationLimit=50  LowerSaturationLimit=-1000
  Vcq : Scope
  Iline_DQ : Outport  VectorParamsAs1DForOutWhenUnconnected=off
  Vpcc_DQ : Outport  Port=2  VectorParamsAs1DForOutWhenUnconnected=off
  wires:
  Mux2/1 -> Iline_DQ/1
  Iinv_DQ/1 -> Demux2/1
  Demux2/2 -> Sum14/1
  Demux2/1 -> Sum15/2
  [wL] -> Product2/1, Product1/1
  Product1/1 -> Sum1/3
  4/1 -> Iline_Q_int/1
  3/1 -> Sum1/4
  Product2/1 -> Sum8/3
  2/1 -> Sum8/4
  Sum8/1 -> 1/1
  Iline_Q_int/1 -> 3/1, Product2/2, Iq/1, [Iq], Mux2/2
  Iline_D_int/1 -> Mux2/1, 2/1, Id/1, Product1/2, [Id]
  1/1 -> Iline_D_int/1
  Sum1/1 -> 4/1
  [Vpcc_D] -> Sum8/1
  [Vpcc_Q] -> Sum1/1
  omega_ref/1 -> 8/1, 7/1
  7/1 -> [wL]
  9/1 -> Vcfd_int/1
  Sum14/1 -> 10/1
  [wcs] -> Product8/1, Product7/1
  [Id] -> Sum15/3
  Vcfq_int/1 -> Mux1/2, [Vpcc_Q], Product7/2, Vcq/1
  Product7/1 -> Sum15/1
  [Iq] -> Sum14/2
  10/1 -> Vcfq_int/1
  Sum15/1 -> 9/1
  Product8/1 -> Sum14/3
  8/1 -> [wcs]
  Vcfd_int/1 -> Product8/2, Mux1/1, [Vpcc_D], Vcd/1
  Mux1/1 -> Vpcc_DQ/1
  Demux1/1 -> Sum8/2
  Demux1/2 -> Sum1/2
  "VsDQ "/1 -> Demux1/1

== system simli_wdc_wWT/ROCOF test1 ==
  Clock : Clock
  Constant4 : Constant  Value=0
  Constant5 : Constant
  Ramp : simulink/Sources/Ramp  slope=rocof_slope  start=Trocof_start  InitialOutput=0
  Sample and Hold : spsSampleandHoldLib/Sample and Hold  ic=0  Ts=0
      settings: LibrarySourceBlock=|
      | sps_lib/Control/Sample and
      | Hold
  Switch : Switch  Criteria=u2 > Threshold  Threshold=Trocof_start  SaturateOnIntegerOverflow=off  InputSameDT=off
  Switch1 : Switch  Threshold=Trocof_end  SaturateOnIntegerOverflow=off  InputSameDT=off
  Outport : Outport
  wires:
  Clock/1 -> Switch/2, Switch1/2
  Constant4/1 -> Switch/3, Switch1/1
  Sample and Hold/1 -> Outport/1
  Ramp/1 -> Switch/1
  Constant5/1 -> Switch1/3
  Switch/1 -> Sample and Hold/1
  Switch1/1 -> Sample and Hold/2
